simulink model "simscape_robot_delta_v8_4"  (R2024b)
settings: Solver=ode23t  StartTime=0.0  StopTime=20.0  FixedStep=1e-3  RelTol=1e-3
model workspace (MAT data in the model file):
  kd1 = 14
  kd2 = 13.6
  kd3 = 37.9
  ki1 = 39
  ki2 = 36
  ki3 = 11.6
  kp1 = 12.6
  kp2 = 12.2
  kp3 = 14.4
values from neighbouring files (symbols this model uses):
  N = floor(size(err,1)/window)    [grafica_error.m]
undefined symbols (not defined in the file or in its folder): X, Y, Z
libraries: sm_lib x74, nesl_utility x10
(part 1 of 3)
settings Model: Creator=rodri  LastModifiedBy=rodri
settings SolverCC: SolverResetMethod=Robust  ODENIntegrationMethod=ode8

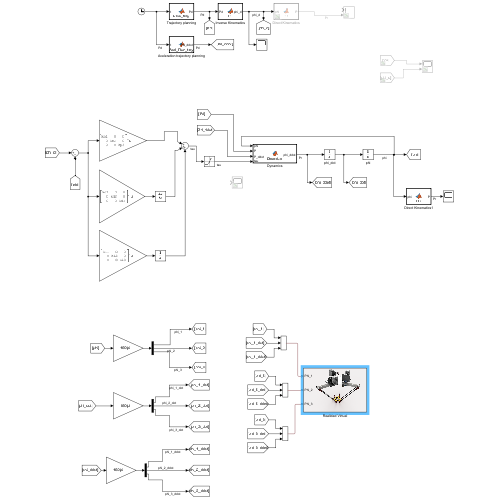
[thumbnail: Simulink's stored preview of the top-level diagram]
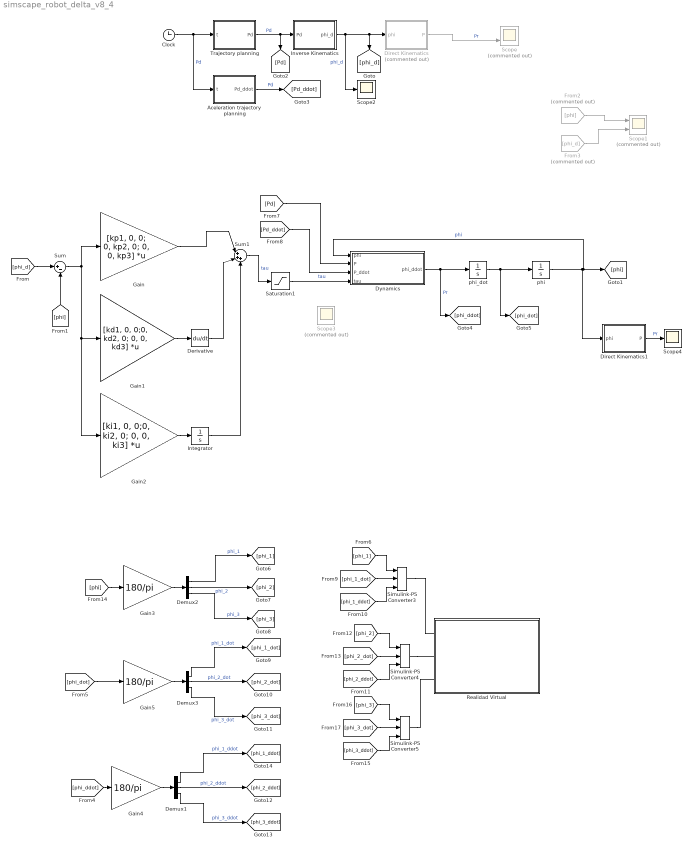
== system simscape_robot_delta_v8_4 ==
  Aceleration trajectory planning : MATLAB Function  TreatAsAtomicUnit=on
  Clock : Clock
  Demux1 : Demux  Outputs=3
  Demux2 : Demux  Outputs=3
  Demux3 : Demux  Outputs=3
  Derivative : Derivative
  Direct Kinematics : MATLAB Function  Commented=on  TreatAsAtomicUnit=on
  Direct Kinematics1 : MATLAB Function  TreatAsAtomicUnit=on
  Dynamics : MATLAB Function  TreatAsAtomicUnit=on
  From2 : From  Commented=on  GotoTag=phi
  From3 : From  Commented=on  GotoTag=phi_d
  Gain : Gain  Gain=[kp1, 0, 0; 0, kp2, 0; 0, 0, kp3]  Multiplication=Matrix(K*u)
  Gain1 : Gain  Gain=[kd1, 0, 0;0, kd2, 0; 0, 0, kd3]  Multiplication=Matrix(K*u)
  Gain2 : Gain  Gain=[ki1, 0, 0;0, ki2, 0; 0, 0, ki3]  Multiplication=Matrix(K*u)
  Gain3 : Gain  Gain=180/pi
  Gain4 : Gain  Gain=180/pi
  Gain5 : Gain  Gain=180/pi
  Integrator : Integrator  InitialCondition=[0;0;0]
  Inverse Kinematics : MATLAB Function  TreatAsAtomicUnit=on
  Realidad Virtual : Subsystem
      mask Display: image('robot_delta_azucena.png');
  Saturation1 : Saturate  UpperLimit=28  LowerLimit=-28
  Scope : Scope  Commented=on  NumInputPorts=2
  Scope1 : Scope  Commented=on  NumInputPorts=2
  Scope2 : Scope
  Scope3 : Scope  Commented=on
  Scope4 : Scope
  Simulink-PS Converter3 : nesl_utility/Simulink-PS Converter  PhysicalDomain=network_engine_domain  SubClassName=ps_input  LeftPortType=input  RightPortType=output  PseudoPeriodic=off  Frequencies=[]  NoiseDistribution=none  NoiseParameters=[]  Unit=deg  AffineConversion=off  FilteringAndDerivatives=provide  SimscapeFilterOrder=1  InputFilterTimeConstant=0.001  UdotUserProvided=2
  Simulink-PS Converter4 : nesl_utility/Simulink-PS Converter  PhysicalDomain=network_engine_domain  SubClassName=ps_input  LeftPortType=input  RightPortType=output  PseudoPeriodic=off  Frequencies=[]  NoiseDistribution=none  NoiseParameters=[]  Unit=deg  AffineConversion=off  FilteringAndDerivatives=provide  SimscapeFilterOrder=1  InputFilterTimeConstant=0.001  UdotUserProvided=2
  Simulink-PS Converter5 : nesl_utility/Simulink-PS Converter  PhysicalDomain=network_engine_domain  SubClassName=ps_input  LeftPortType=input  RightPortType=output  PseudoPeriodic=off  Frequencies=[]  NoiseDistribution=none  NoiseParameters=[]  Unit=deg  AffineConversion=off  FilteringAndDerivatives=provide  SimscapeFilterOrder=1  InputFilterTimeConstant=0.001  UdotUserProvided=2
  Sum : Sum  Inputs=|+-
  Sum1 : Sum  Inputs=|+++
  Trajectory planning : MATLAB Function  TreatAsAtomicUnit=on
  phi : Integrator  InitialCondition=[0;0;0]
  phi_dot : Integrator  InitialCondition=[0;0;0]
  wires:
  Sum/1 -> Gain2/1, Gain1/1, Gain/1
  Gain/1 -> Sum1/1
  Derivative/1 -> Sum1/2
  [Pd] -> Dynamics/2(P)
  Clock/1 -> Aceleration trajectory planning/1(t), Trajectory planning/1(t)  "Pd"
  phi/1 -> Direct Kinematics1/1(phi), Dynamics/1(phi), [phi]  "phi"
  Direct Kinematics/1(P) -> Scope/2  "Pr"
  Integrator/1 -> Sum1/3
  [Pd_ddot] -> Dynamics/3(P_ddot)
  Gain1/1 -> Derivative/1
  [phi_d] -> Sum/1
  Trajectory planning/1(Pd) -> Inverse Kinematics/1(Pd), [Pd]  "Pd"
  From3/1 -> Scope1/2
  Dynamics/1(phi_ddot) -> [phi_ddot], phi_dot/1  "Pr"
  Gain2/1 -> Integrator/1
  phi_dot/1 -> [phi_dot], phi/1
  Inverse Kinematics/1(phi_d) -> Scope2/1, [phi_d], Direct Kinematics/1(phi)  "phi_d"
  Aceleration trajectory planning/1(Pd_ddot) -> [Pd_ddot]  "Pd"
  From2/1 -> Scope1/1
  [phi] -> Sum/2
  Demux2/1 -> [phi_1]  "phi_1"
  [phi] -> Gain3/1
  Gain3/1 -> Demux2/1
  Demux2/3 -> [phi_3]  "phi_3"
  Demux2/2 -> [phi_2]  "phi_2"
  Demux1/3 -> [phi_3_ddot]  "phi_3_ddot"
  Demux1/2 -> [phi_2_ddot]  "phi_2_ddot"
  Demux1/1 -> [phi_1_ddot]  "phi_1_ddot"
  Gain4/1 -> Demux1/1
  [phi_ddot] -> Gain4/1
  [phi_dot] -> Gain5/1
  Demux3/1 -> [phi_1_dot]  "phi_1_dot"
  Gain5/1 -> Demux3/1
  Demux3/2 -> [phi_2_dot]  "phi_2_dot"
  Demux3/3 -> [phi_3_dot]  "phi_3_dot"
  [phi_1] -> Simulink-PS Converter3/1
  [phi_1_dot] -> Simulink-PS Converter3/2
  [phi_1_ddot] -> Simulink-PS Converter3/3
  [phi_2_dot] -> Simulink-PS Converter4/2
  [phi_2] -> Simulink-PS Converter4/1
  [phi_2_ddot] -> Simulink-PS Converter4/3
  [phi_3_dot] -> Simulink-PS Converter5/2
  [phi_3] -> Simulink-PS Converter5/1
  [phi_3_ddot] -> Simulink-PS Converter5/3
  Direct Kinematics1/1(P) -> Scope4/1  "Pr"
  Saturation1/1 -> Dynamics/4(tau)  "tau"
  Sum1/1 -> Saturation1/1  "tau"
  connections:
  Simulink-PS Converter3/RConn1 -- Realidad Virtual/LConn1
  Simulink-PS Converter4/RConn1 -- Realidad Virtual/LConn2
  Simulink-PS Converter5/RConn1 -- Realidad Virtual/LConn3
